simulink model "drunk"  (Simulink 10.3)
settings: Solver=ode1  StartTime=0.0  StopTime=30  FixedStep=0.01  RelTol=1e-3  EnableMultiTasking=on
undefined symbols (not defined in the file): HIL, Host
libraries: quarc_library x9, pid_lib x1
settings Model: Creator=drmadill  LastModifiedBy=Rohan  SimulationMode=external  ExtModeTrigDuration=2
settings SolverCC: PositivePriorityOrder=on
settings DataIOCC: LimitDataPoints=on
settings OptimizationCC: LifeSpan=auto
settings DebuggingCC: SolverPrmCheckMsg=warning
settings HardwareCC: ProdLargestAtomicInteger=Long  ProdLargestAtomicFloat=Double  ProdIntDivRoundTo=Zero  ProdEndianess=LittleEndian  ProdHWDeviceType=ARM Compatible->ARM Cortex
settings RTWCC: Description=QUARC Linux Raspberry Pi 3 Target (QBot 2e) Using Toolchain  SystemTargetFile=quarc_linux_pi_3.tlc  TemplateMakefile=quarc_default_tmf  Toolchain=QUARC linux_pi_3 | gmake (64-bit Windows)  BuildConfiguration=Faster Runs
settings STFCustomTargetCC: ConcurrentExecutionCompliant=on  UseToolchainInfoCompliant=on  SystemTargetFile=quarc_linux_pi_3.tlc
settings GRTTargetCC: ParMdlRefBuildCompliant=off  CompOptLevelCompliant=off  MatFileLogging=off  CPPClassGenCompliant=off  ExtMode=on  ExtModeMexFile=quarc_comm  ExtModeMexArgs='-w -d /tmp -uri %u', 'tcpip://192.168.2.28:17001'
settings ConfigComp: CovSFcnEnable=off

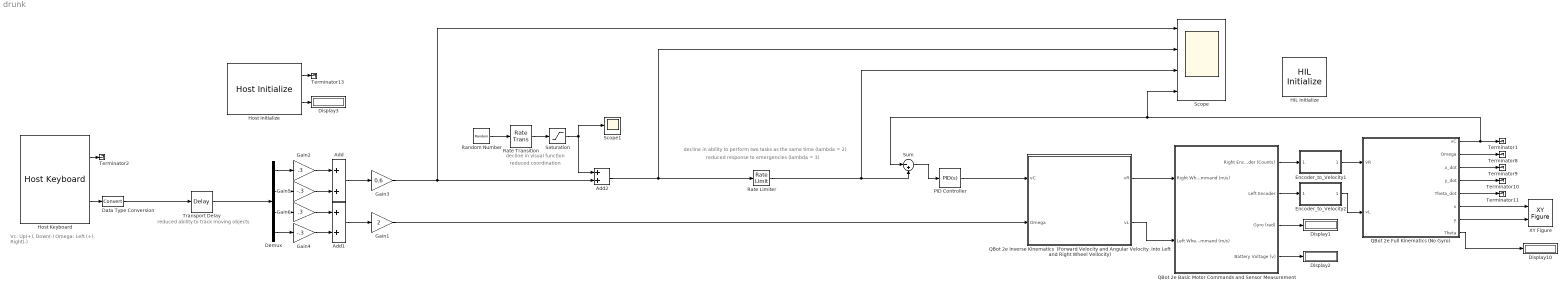
== system drunk ==
  note: Vc: Up(+), Down(-)
      | Omega: Left (+), Right(-)
  note: decline in visual function
  note: reduced coordination
  note: reduced ability to track moving objects
  note: reduced response to emergencies (lambda = 3)
  note: decline in ability to perform two tasks as the same time (lambda = 2)
  Add : Sum
  Add1 : Sum
  Add2 : Sum
  Data Type Conversion : DataTypeConversion
  Demux : Demux
  Display{1..3,10} (4 alike) : Display
  Encoder_to_Velocity1 : Subsystem
  Encoder_to_Velocity2 : Subsystem
  Gain1 : Gain  Gain=2
  Gain2 : Gain  Gain=.3
  Gain3 : Gain  Gain=0.6
  Gain4 : Gain  Gain=-.3
  Gain5 : Gain  Gain=-.3
  Gain6 : Gain  Gain=.3
  HIL Initialize : quarc_library/Data Acquisition/Generic/Configuration/HIL Initialize  Priority=-99  object_name=HIL-1  board_type=qbot2e  board_number=0  board_options=pwm0_en=1;pwm0_pin=12;pwm1_en=1;pwm1_pin=13;  exclusive=off  active=off  hardware_clocks=[]  clock_modes=[]  initial_clock_frequencies=[]  set_clock_params_at_start=off  set_clock_params_at_switch_in=off  set_clock_frequencies_at_start=off  set_clock_frequencies_at_switch_in=off  analog_input_channels=[0:5]  analog_input_configurations=[]  analog_input_maximums=[16.5 3.3 3.3 3.3 3.3 3.3]  analog_input_minimums=[0 0 0 0 0 0]  set_analog_input_params_at_start=off  set_analog_input_params_at_switch_in=off  analog_output_channels=[]  analog_output_maximums=[]  analog_output_minimums=[]  initial_analog_outputs=[]  final_analog_outputs=[]  watchdog_analog_outputs=[]  set_analog_output_params_at_start=off  set_analog_output_params_at_switch_in=off  set_analog_outputs_at_start=off  set_analog_outputs_at_switch_in=off  set_analog_outputs_at_terminate=off  set_analog_outputs_at_switch_out=off  set_analog_outputs_on_watchdog=off  digital_input_channels=[28:58]  digital_output_channels=[28:31]  digital_output_configuration=[]  initial_digital_outputs=[0]  final_digital_outputs=[0]  watchdog_digital_outputs=[]  set_digital_output_params_at_start=off  set_digital_output_params_at_switch_in=off  set_digital_outputs_at_start=on  set_digital_outputs_at_switch_in=off  set_digital_outputs_at_terminate=on  set_digital_outputs_at_switch_out=off  set_digital_outputs_on_watchdog=off  encoder_channels=[0:1]  quadrature=[4]  encoder_filter_frequency=[]  initial_encoder_counts=[0]  set_encoder_params_at_start=on  set_encoder_params_at_switch_in=off  set_encoder_counts_at_start=on  set_encoder_counts_at_switch_in=off  pwm_channels=[0:1]  pwm_modes=0  pwm_frequency=100e6 / 4095  pwm_configuration=[0]  pwm_alignment=[0]  pwm_polarity=[1]  pwm_leading_deadband=[]  pwm_trailing_deadband=[]  initial_pwm_outputs=[0]  final_pwm_outputs=[0]  watchdog_pwm_outputs=[]  set_pwm_params_at_start=on  set_pwm_params_at_switch_in=off  set_pwm_outputs_at_start=on  set_pwm_outputs_at_switch_in=off  set_pwm_outputs_at_terminate=on  set_pwm_outputs_at_switch_out=off  set_pwm_outputs_on_watchdog=off  other_output_channels=[2000:2001 14000 16000]  initial_other_outputs=[0 0 0 7]  final_other_outputs=[0 0 0 7]  watchdog_other_outputs=[]  set_other_outputs_at_start=on  set_other_outputs_at_switch_in=off  set_other_outputs_at_terminate=on  set_other_outputs_at_switch_out=off  set_other_outputs_on_watchdog=off
  Host Initialize : quarc_library/Devices/Peripherals/Host/Host Initialize  object_name=Host-1  uri_source=Use external mode communications  uri=tcpip://192.168.2.104:17001  apply_uri_to_all_configs=on  send_buffer_size=1000  receive_buffer_size=1000  thread_priority=0  run_client=on  use_window=off  window_position=[]  sample_time=qc_get_step_size  active=on
      settings: SourceProductName=QUARC Targets
  Host Keyboard : quarc_library/Devices/Peripherals/Host/Host Keyboard  object_name=Host-1  virtual_key="[38  40  37  39]"  sample_time=qc_get_step_size  enabled=on  debug_mode=off
      settings: SourceProductName=QUARC Targets
  PID Controller : pid_lib/PID Controller  Controller=PID  Form=Parallel  TimeDomain=Continuous-time  UseExternalTs=off  SampleTime=-1  IntegratorMethod=Forward Euler  FilterMethod=Forward Euler  ControllerParametersSource=internal  P=1  I=2.5  D=0  UseFilter=on  N=100  TunerSelectOption=Transfer Function Based (PID Tuner App)  InitialConditionSource=internal  InitialConditionForIntegrator=0  InitialConditionForFilter=0  DifferentiatorICPrevScaledInput=0  ExternalReset=none  TrackingMode=off  Kt=1  LimitOutput=off  SatLimitsSource=internal  UpperSaturationLimit=inf  LowerSaturationLimit=-inf  LinearizeAsGain=on  AntiWindupMode=none  Kb=1  POutMin=[]  POutMax=[]  IOutMin=[]  IOutMax=[]  DOutMin=[]  DOutMax=[]  NOutMin=[]  NOutMax=[]  SumOutMin=[]  SumOutMax=[]  SaturationOutMin=[]  SaturationOutMax=[]  PParamMin=[]  PParamMax=[]  IParamMin=[]  IParamMax=[]  DParamMin=[]  DParamMax=[]  NParamMin=[]  NParamMax=[]  KbParamMin=[]  KbParamMax=[]  KtParamMin=[]  KtParamMax=[]  KbOutMin=[]  KbOutMax=[]  KtOutMin=[]  KtOutMax=[]  IntegratorOutMin=[]  IntegratorOutMax=[]  FilterOutMin=[]  FilterOutMax=[]  SumI1OutMin=[]  SumI1OutMax=[]  SumI2OutMin=[]  SumI2OutMax=[]  SumI3OutMin=[]  SumI3OutMax=[]  SumI4OutMin=[]  SumI4OutMax=[]  SumDOutMin=[]  SumDOutMax=[]  DifferentiatorOutMin=[]  DifferentiatorOutMax=[]  FilterDiffOutCoefMin=[]  FilterDiffOutCoefMax=[]  ReciprocalOutMin=[]  ReciprocalOutMax=[]  SumDenOutMin=[]  SumDenOutMax=[]  SumNumOutMin=[]  SumNumOutMax=[]  DivideOutMin=[]  DivideOutMax=[]  UdiffTsProdOutMin=[]  UdiffTsProdOutMax=[]  NTsProdOutMin=[]  NTsProdOutMax=[]  UintegralTsProdOutMin=[]  UintegralTsProdOutMax=[]  UngainTsProdOutMin=[]  UngainTsProdOutMax=[]  IntegratorContinuousStateAttributes=''  IntegratorStateMustResolveToSignalObject=off  IntegratorRTWStateStorageClass=Auto  FilterContinuousStateAttributes=''  FilterStateMustResolveToSignalObject=off  FilterRTWStateStorageClass=Auto  ParallelPVariant=InternalParameters  IdealPVariant=Disabled  IVariant=InternalParameters  DVariant=InternalParameters  IntegratorVariant=Continuous  SatVariant=Disabled  AWVariant=Passthrough  PCopyVariant=Disabled  TRVariant=Disabled  FdbkBlocksVariant=Forward  IdealPFdbkVariant=Disabled  SatFdbkVariant=Disabled  DerivativeFilterVariant=ContFilter  NVariant=InternalParameters  NCopyVariant=Disabled  FilterICVariant=InternalICsFilter  IntegratorICVariant=InternalICs  ExternalResetVariant=Disabled  TRSumVariant=Passthrough  SumFdbkVariant=Disabled  SumVariant=Sum_PID  TsampFilterVariant=InternalTs  TsampNgainVariant=Passthrough  TsampIntegralVariant=Passthrough  ExternalSaturationOutDataTypeStr=Inherit: Same as second input
  QBot 2e Basic Motor Commands and Sensor Measurement : Subsystem
  QBot 2e Full Kinematics (No Gyro) : Subsystem
  QBot 2e Inverse Kinematics  (Forward Velocity and Angular Velocity  into Left and Right Wheel Vellocity) : Subsystem
  Random Number : RandomNumber  Variance=.01  SampleTime=1
  Rate Limiter : RateLimiter  SampleTimeMode=inherited
  Rate Transition : RateTransition
  Saturation : Saturate  UpperLimit=.1  LowerLimit=-.1
  Scope : Scope  NumInputPorts=4
  Scope1 : Scope
  Sum : Sum  Inputs=|-+
  Terminator{1..2,8..11,13} (7 alike) : Terminator
  Transport Delay : TransportDelay  DelayTime=.12
  XY Figure : quarc_library/Sinks/Figures/XY Figure  figure_mode=Use figure window  figure_tag=figure1  axes_tag=axes1  plot_mode=Time-based  minimum_x=-1  maximum_x=1  minimum_y=-1  maximum_y=1  buffer_size=1000  update_rate=100  initial_position="672  171  710  615"  initial_visibility=off  sample_time=-1
      settings: SourceProductName=QUARC Targets
  wires:
  Host Initialize/2 -> Display3/1
  Host Initialize/1 -> Terminator13/1
  QBot 2e Basic Motor Commands and Sensor Measurement/2(Left Encoder) -> Encoder_to_Velocity2/1(Encoder)
  QBot 2e Full Kinematics (No Gyro)/8(Theta) -> Display10/1
  QBot 2e Full Kinematics (No Gyro)/7(y) -> XY Figure/2
  QBot 2e Full Kinematics (No Gyro)/6(x) -> XY Figure/1
  Encoder_to_Velocity1/1(Velocity) -> QBot 2e Full Kinematics (No Gyro)/1(vR)
  Encoder_to_Velocity2/1(Velocity) -> QBot 2e Full Kinematics (No Gyro)/2(vL)
  QBot 2e Inverse Kinematics  (Forward Velocity and Angular Velocity  into Left and Right Wheel Vellocity)/1(vR) -> QBot 2e Basic Motor Commands and Sensor Measurement/1(Right Wheel Command (m/s))
  Gain3/1 -> Scope/1, Add2/2
  QBot 2e Full Kinematics (No Gyro)/2(Omega) -> Terminator8/1
  QBot 2e Full Kinematics (No Gyro)/3(x_dot) -> Terminator9/1
  QBot 2e Full Kinematics (No Gyro)/4(y_dot) -> Terminator10/1
  QBot 2e Full Kinematics (No Gyro)/5(Theta_dot) -> Terminator11/1
  Host Keyboard/2 -> Data Type Conversion/1
  Demux/1 -> Gain2/1
  Demux/4 -> Gain4/1
  Gain2/1 -> Add/1
  Add/1 -> Gain3/1
  Demux/2 -> Gain5/1
  Demux/3 -> Gain6/1
  Add1/1 -> Gain1/1
  Data Type Conversion/1 -> Transport Delay/1
  Gain5/1 -> Add/2
  Gain6/1 -> Add1/1
  Gain4/1 -> Add1/2
  QBot 2e Full Kinematics (No Gyro)/1(vC) -> Sum/1, Scope/4, Terminator1/1
  Host Keyboard/1 -> Terminator2/1
  Gain1/1 -> QBot 2e Inverse Kinematics  (Forward Velocity and Angular Velocity  into Left and Right Wheel Vellocity)/2(Omega)
  QBot 2e Inverse Kinematics  (Forward Velocity and Angular Velocity  into Left and Right Wheel Vellocity)/2(vL) -> QBot 2e Basic Motor Commands and Sensor Measurement/2(Left Wheel Command (m/s))
  QBot 2e Basic Motor Commands and Sensor Measurement/1(Right Encoder (Counts)) -> Encoder_to_Velocity1/1(Encoder)
  QBot 2e Basic Motor Commands and Sensor Measurement/3(Gyro (rad)) -> Display1/1
  QBot 2e Basic Motor Commands and Sensor Measurement/4(Battery Voltage (v)) -> Display2/1
  Transport Delay/1 -> Demux/1
  Random Number/1 -> Rate Transition/1
  Saturation/1 -> Add2/1, Scope1/1
  Rate Transition/1 -> Saturation/1
  PID Controller/1 -> QBot 2e Inverse Kinematics  (Forward Velocity and Angular Velocity  into Left and Right Wheel Vellocity)/1(vC)
  Sum/1 -> PID Controller/1
  Add2/1 -> Rate Limiter/1, Scope/2
  Rate Limiter/1 -> Scope/3, Sum/2

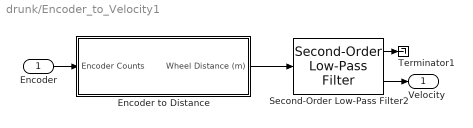
== system drunk/Encoder_to_Velocity1 ==
  Encoder : Inport
  Encoder to Distance : Subsystem
  Second-Order Low-Pass Filter2 : quarc_library/Continuous/Second-Order Low-Pass Filter  params_source=Internal (dialog parameters)  input_width=10  input_zeta=1  input_init=0
  Terminator1 : Terminator
  Velocity : Outport
  wires:
  Second-Order Low-Pass Filter2/2 -> Velocity/1
  Encoder/1 -> Encoder to Distance/1(Encoder Counts)
  Encoder to Distance/1(Wheel Distance (m)) -> Second-Order Low-Pass Filter2/1
  Second-Order Low-Pass Filter2/1 -> Terminator1/1

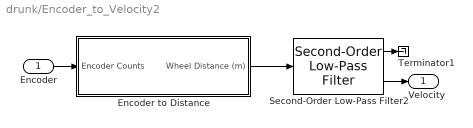
== system drunk/Encoder_to_Velocity2 ==
  Encoder : Inport
  Encoder to Distance : Subsystem
  Second-Order Low-Pass Filter2 : quarc_library/Continuous/Second-Order Low-Pass Filter  params_source=Internal (dialog parameters)  input_width=10  input_zeta=1  input_init=0
  Terminator1 : Terminator
  Velocity : Outport
  wires:
  Second-Order Low-Pass Filter2/1 -> Terminator1/1
  Encoder to Distance/1(Wheel Distance (m)) -> Second-Order Low-Pass Filter2/1
  Encoder/1 -> Encoder to Distance/1(Encoder Counts)
  Second-Order Low-Pass Filter2/2 -> Velocity/1

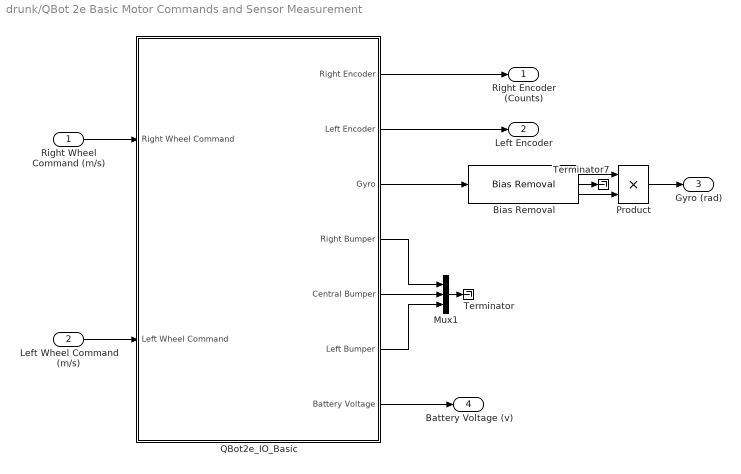
== system drunk/QBot 2e Basic Motor Commands and Sensor Measurement ==
  Right Wheel Command (m/s) : Inport
  Left Wheel Command (m/s) : Inport  Port=2
  Bias Removal : quarc_library/Discrete/Bias Removal  start_time=3  end_time=4  switch_id=0  sample_time=qc_get_step_size
      settings: SourceProductName=QUARC Targets
  Mux1 : Mux  Inputs=3
  Product : Product  RndMeth=Zero
  QBot2e_IO_Basic : Subsystem
  Terminator : Terminator
  Terminator7 : Terminator
  Right Encoder (Counts) : Outport
  Left Encoder : Outport  Port=2
  Gyro (rad) : Outport  Port=3
  Battery Voltage (v) : Outport  Port=4
  wires:
  QBot2e_IO_Basic/4(Right Bumper) -> Mux1/1
  QBot2e_IO_Basic/5(Central Bumper) -> Mux1/2
  QBot2e_IO_Basic/6(Left Bumper) -> Mux1/3
  Right Wheel Command (m/s)/1 -> QBot2e_IO_Basic/1(Right Wheel Command)
  Left Wheel Command (m/s)/1 -> QBot2e_IO_Basic/2(Left Wheel Command)
  QBot2e_IO_Basic/1(Right Encoder) -> Right Encoder (Counts)/1
  QBot2e_IO_Basic/2(Left Encoder) -> Left Encoder/1
  QBot2e_IO_Basic/7(Battery Voltage) -> Battery Voltage (v)/1
  Bias Removal/2 -> Terminator7/1
  Bias Removal/1 -> Product/1
  Bias Removal/3 -> Product/2
  Product/1 -> Gyro (rad)/1
  QBot2e_IO_Basic/3(Gyro) -> Bias Removal/1
  Mux1/1 -> Terminator/1

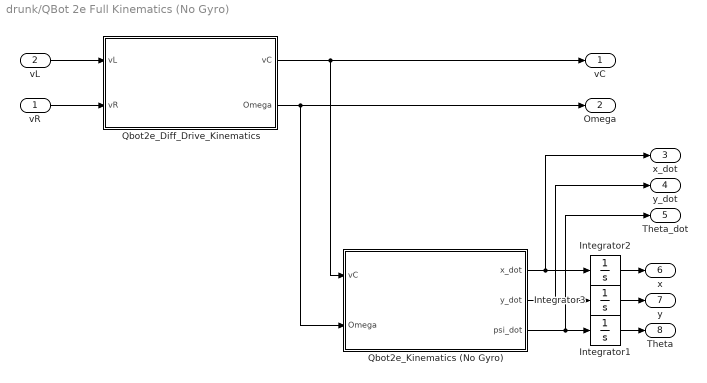
== system drunk/QBot 2e Full Kinematics (No Gyro) ==
  vR : Inport
  vL : Inport  Port=2
  Integrator1 : Integrator
  Integrator2 : Integrator
  Integrator3 : Integrator
  Qbot2e_Diff_Drive_Kinematics : Subsystem
  Qbot2e_Kinematics (No Gyro) : Subsystem
  vC : Outport
  Omega : Outport  Port=2
  x_dot : Outport  Port=3
  y_dot : Outport  Port=4
  Theta_dot : Outport  Port=5
  x : Outport  Port=6
  y : Outport  Port=7
  Theta : Outport  Port=8
  wires:
  Qbot2e_Diff_Drive_Kinematics/2(Omega) -> Omega/1, Qbot2e_Kinematics (No Gyro)/2(Omega)
  Integrator3/1 -> y/1
  Integrator2/1 -> x/1
  vR/1 -> Qbot2e_Diff_Drive_Kinematics/2(vR)
  vL/1 -> Qbot2e_Diff_Drive_Kinematics/1(vL)
  Qbot2e_Diff_Drive_Kinematics/1(vC) -> vC/1, Qbot2e_Kinematics (No Gyro)/1(vC)
  Qbot2e_Kinematics (No Gyro)/2(y_dot) -> Integrator3/1, y_dot/1
  Qbot2e_Kinematics (No Gyro)/1(x_dot) -> Integrator2/1, x_dot/1
  Qbot2e_Kinematics (No Gyro)/3(psi_dot) -> Integrator1/1, Theta_dot/1
  Integrator1/1 -> Theta/1

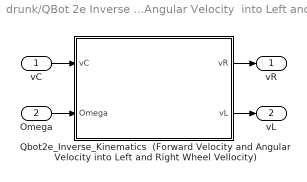
== system drunk/QBot 2e Inverse Kinematics  (Forward Velocity and Angular Velocity  into Left and Right Wheel Vellocity) ==
  vC : Inport
  Omega : Inport  Port=2
  Qbot2e_Inverse_Kinematics  (Forward Velocity and Angular Velocity into Left and Right Wheel Vellocity) : MATLAB Function  TreatAsAtomicUnit=on
  vR : Outport
  vL : Outport  Port=2
  wires:
  vC/1 -> Qbot2e_Inverse_Kinematics  (Forward Velocity and Angular Velocity into Left and Right Wheel Vellocity)/1(vC)
  Qbot2e_Inverse_Kinematics  (Forward Velocity and Angular Velocity into Left and Right Wheel Vellocity)/1(vR) -> vR/1
  Omega/1 -> Qbot2e_Inverse_Kinematics  (Forward Velocity and Angular Velocity into Left and Right Wheel Vellocity)/2(Omega)
  Qbot2e_Inverse_Kinematics  (Forward Velocity and Angular Velocity into Left and Right Wheel Vellocity)/2(vL) -> vL/1

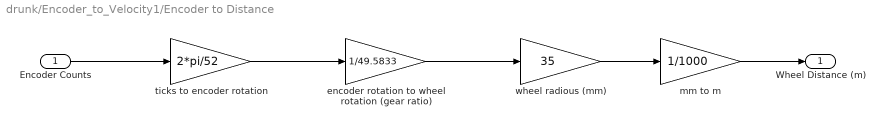
== system drunk/Encoder_to_Velocity1/Encoder to Distance ==
  Encoder Counts : Inport
  " encoder rotation to wheel rotation (gear ratio)" : Gain  Gain=1/49.5833
  mm to m : Gain  Gain=1/1000
  ticks to encoder rotation : Gain  Gain=2*pi/52
  wheel radious (mm) : Gain  Gain=35
  Wheel Distance (m) : Outport
  wires:
  mm to m/1 -> Wheel Distance (m)/1
  wheel radious (mm)/1 -> mm to m/1
  " encoder rotation to wheel rotation (gear ratio)"/1 -> wheel radious (mm)/1
  ticks to encoder rotation/1 -> " encoder rotation to wheel rotation (gear ratio)"/1
  Encoder Counts/1 -> ticks to encoder rotation/1

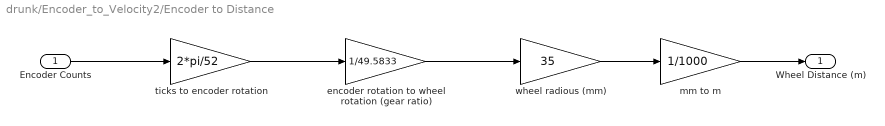
== system drunk/Encoder_to_Velocity2/Encoder to Distance ==
  Encoder Counts : Inport
  " encoder rotation to wheel rotation (gear ratio)" : Gain  Gain=1/49.5833
  mm to m : Gain  Gain=1/1000
  ticks to encoder rotation : Gain  Gain=2*pi/52
  wheel radious (mm) : Gain  Gain=35
  Wheel Distance (m) : Outport
  wires:
  Encoder Counts/1 -> ticks to encoder rotation/1
  ticks to encoder rotation/1 -> " encoder rotation to wheel rotation (gear ratio)"/1
  " encoder rotation to wheel rotation (gear ratio)"/1 -> wheel radious (mm)/1
  wheel radious (mm)/1 -> mm to m/1
  mm to m/1 -> Wheel Distance (m)/1

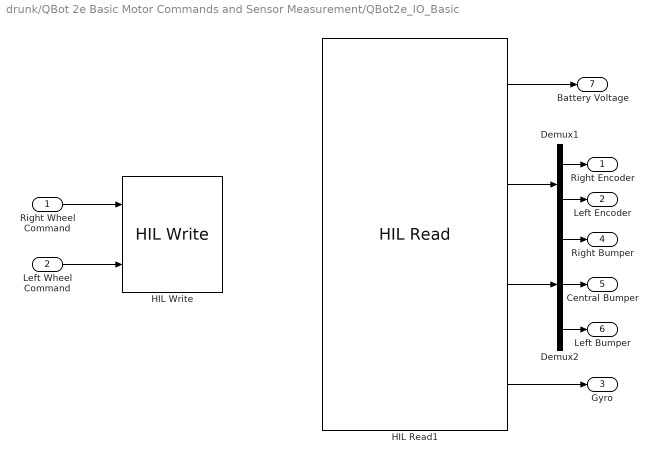
== system drunk/QBot 2e Basic Motor Commands and Sensor Measurement/QBot2e_IO_Basic ==
  Right Wheel Command : Inport
  Left Wheel Command : Inport  Port=2
  Demux1 : Demux  Outputs=2
  Demux2 : Demux  Outputs=3
  HIL Read1 : quarc_library/Data Acquisition/Generic/Immediate I//O/HIL Read  object_name=HIL-1  analog_channels=[0]  encoder_channels=[0:1]  digital_channels=[28:30]  other_channels=[1002]  sample_time=qc_get_step_size  active=on  vector_output=on  data_type_mode=Inherit via back propagation  encoder_data_type=double  digital_data_type=boolean
  HIL Write : quarc_library/Data Acquisition/Generic/Immediate I//O/HIL Write  object_name=HIL-1  analog_channels=[]  pwm_channels=[]  digital_channels=[]  other_channels=[2000:2001]  sample_time=-1  active=on  vector_input=off
  Right Encoder : Outport
  Left Encoder : Outport  Port=2
  Gyro : Outport  Port=3
  Right Bumper : Outport  Port=4
  Central Bumper : Outport  Port=5
  Left Bumper : Outport  Port=6
  Battery Voltage : Outport  Port=7
  wires:
  HIL Read1/1 -> Battery Voltage/1
  HIL Read1/3 -> Demux2/1
  HIL Read1/4 -> Gyro/1
  Demux1/1 -> Right Encoder/1
  Demux1/2 -> Left Encoder/1
  Right Wheel Command/1 -> HIL Write/1
  Left Wheel Command/1 -> HIL Write/2
  HIL Read1/2 -> Demux1/1
  Demux2/1 -> Right Bumper/1
  Demux2/2 -> Central Bumper/1
  Demux2/3 -> Left Bumper/1

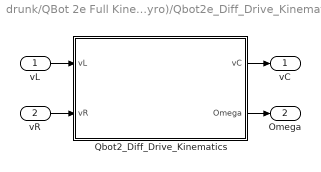
== system drunk/QBot 2e Full Kinematics (No Gyro)/Qbot2e_Diff_Drive_Kinematics ==
  vL : Inport
  vR : Inport  Port=2
  Qbot2_Diff_Drive_Kinematics : MATLAB Function  TreatAsAtomicUnit=on
  vC : Outport
  Omega : Outport  Port=2
  wires:
  Qbot2_Diff_Drive_Kinematics/2(Omega) -> Omega/1
  vR/1 -> Qbot2_Diff_Drive_Kinematics/2(vR)
  Qbot2_Diff_Drive_Kinematics/1(vC) -> vC/1
  vL/1 -> Qbot2_Diff_Drive_Kinematics/1(vL)

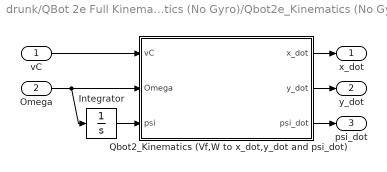
== system drunk/QBot 2e Full Kinematics (No Gyro)/Qbot2e_Kinematics (No Gyro) ==
  vC : Inport
  Omega : Inport  Port=2
  Integrator : Integrator
  Qbot2_Kinematics (Vf,W to x_dot,y_dot and psi_dot) : MATLAB Function  TreatAsAtomicUnit=on
  x_dot : Outport
  y_dot : Outport  Port=2
  psi_dot : Outport  Port=3
  wires:
  Qbot2_Kinematics (Vf,W to x_dot,y_dot and psi_dot)/2(y_dot) -> y_dot/1
  Omega/1 -> Qbot2_Kinematics (Vf,W to x_dot,y_dot and psi_dot)/2(Omega), Integrator/1
  Qbot2_Kinematics (Vf,W to x_dot,y_dot and psi_dot)/1(x_dot) -> x_dot/1
  vC/1 -> Qbot2_Kinematics (Vf,W to x_dot,y_dot and psi_dot)/1(vC)
  Integrator/1 -> Qbot2_Kinematics (Vf,W to x_dot,y_dot and psi_dot)/3(psi)
  Qbot2_Kinematics (Vf,W to x_dot,y_dot and psi_dot)/3(psi_dot) -> psi_dot/1

== matlab function QBot 2e Full Kinematics (No Gyro)/Qbot2e_Diff_Drive_Kinematics/Qbot2_Diff_Drive_Kinematics ==
  data: vL input double; vC output double; vR input double; Omega output double
function [vC,Omega] = fcn(vL,vR)
%#codegen

d= 0.235;

vC=0.5*(vL+vR);
Omega=(1/d)*(vR-vL);

== matlab function QBot 2e Full Kinematics (No Gyro)/Qbot2e_Kinematics (No Gyro)/Qbot2_Kinematics (Vf,W to x_dot,y_dot and psi_dot) ==
  data: vC input double; x_dot output double; Omega input double; y_dot output double; psi input double; psi_dot output double
function [x_dot,y_dot,psi_dot] = fcn(vC,Omega,psi)
%#codegen


x_dot=cos(psi)*vC;
y_dot=sin(psi)*vC;
psi_dot= Omega;

== matlab function QBot 2e Inverse Kinematics (Forward Velocity and Angular Velocity into Left and Right Wheel Vellocity)/Qbot2e_Inverse_Kinematics (Forward Velocity and Angular Velocity into Left and Right Wheel Vellocity) ==
  data: vR output double; vL output double; vC input double; Omega input double
function [vR,vL] = fcn(vC , Omega)
%#codegen

d=0.235; 


vR = vC + Omega*d/2;
vL= vC - Omega*d/2;
